simulink model "model2"  (R2022a)
settings: Solver=VariableStepAuto  StartTime=0.0  StopTime=10.0  RelTol=1e-3
values from neighbouring files (symbols this model uses):
  Gamma_f = 1    [control.m]
  Gamma_g = [0 1 ... (first row only)    [control.m]
  H_f = 1    [control.m]
  K_oc = -H_d/M    [control.m]
  T = 0.2    [config.m]
  xi_f0 = f_0    [control.m]    (also in tasks.m)
  xi_g0 = [0 ... (first row only)    [control.m]
undefined symbols (not defined in the file or in its folder): A, B, L_f, L_g
settings Model: Creator=Vvlad  LastModifiedBy=Vvlad

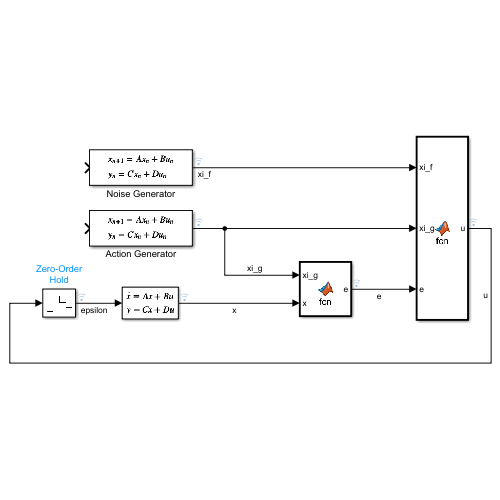
[thumbnail: Simulink's stored preview of the top-level diagram]
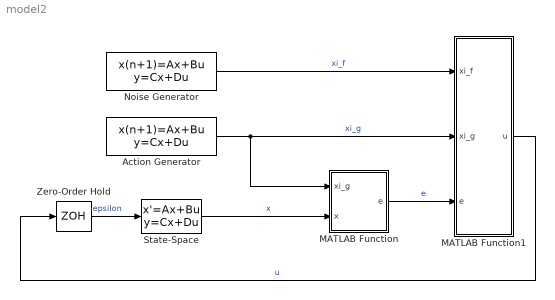
== system model2 ==
  Action Generator : DiscreteStateSpace  A=Gamma_g  B=[0;0]  C=eye(2)  D=[0;0]  InitialCondition=xi_g0  SampleTime=T
  MATLAB Function : MATLAB Function  TreatAsAtomicUnit=on
  MATLAB Function1 : MATLAB Function  TreatAsAtomicUnit=on
  Noise Generator : DiscreteStateSpace  A=Gamma_f  B=0  C=H_f  D=0  InitialCondition=xi_f0  SampleTime=T
  State-Space : StateSpace  A=A  B=B  C=eye(2)  D=[0;0]  InitialCondition=0
  Zero-Order Hold : ZeroOrderHold  SampleTime=-1
  wires:
  State-Space/1 -> MATLAB Function/2(x)  "x"
  Action Generator/1 -> MATLAB Function1/2(xi_g), MATLAB Function/1(xi_g)  "xi_g"
  MATLAB Function/1(e) -> MATLAB Function1/3(e)  "e"
  MATLAB Function1/1(u) -> Zero-Order Hold/1  "u"
  Noise Generator/1 -> MATLAB Function1/1(xi_f)  "xi_f"
  Zero-Order Hold/1 -> State-Space/1  "epsilon"

== matlab function model2/MATLAB Function1 ==
  data: xi_f input; u output; xi_g input; e input; L_f parameter; L_g parameter; K_oc parameter
function u = fcn(xi_f, xi_g, e, L_f, L_g, K_oc)

u =  K_oc*e + L_g*xi_g - L_f*xi_f;

== matlab function model2/MATLAB Function ==
  data: xi_g input; e output; x input; M_g parameter
function e = fcn(xi_g, x, M_g)

e = M_g*xi_g - x;
